simulink model "BlueRov2PID"  (R2025a)
settings: Solver=ode4  StartTime=0.0  StopTime=30  FixedStep=0.001  RelTol=1e-3
settings Model: Creator=oisin  LastModifiedBy=oisin
settings DataIOCC: ReturnWorkspaceOutputsName=PID

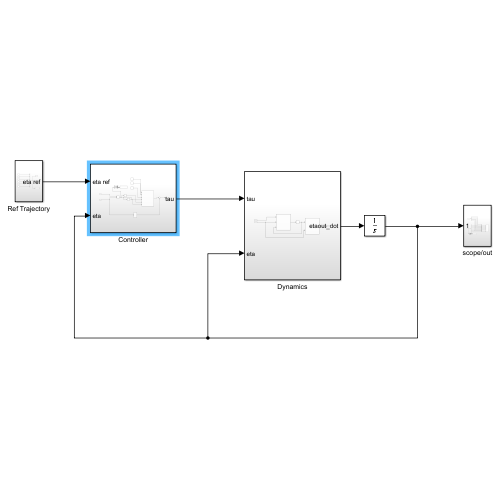
[thumbnail: Simulink's stored preview of the top-level diagram]
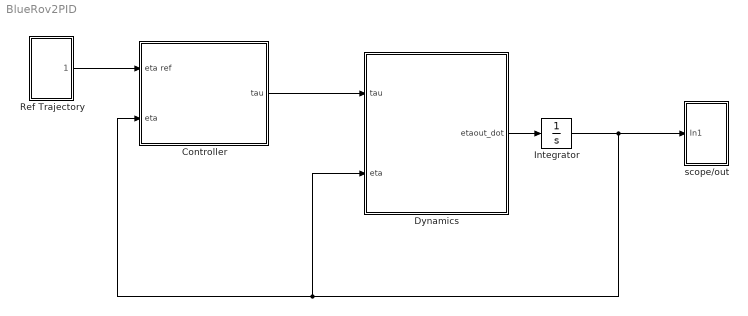
== system BlueRov2PID ==
  Controller : Subsystem
  Dynamics : Subsystem
  Integrator : Integrator  InitialCondition=[10;0;0;0;0;0]
  Ref Trajectory : Subsystem
  scope/out : Subsystem
  wires:
  Ref Trajectory/1(eta ref) -> Controller/1(eta ref)
  Integrator/1 -> Dynamics/2(eta), Controller/2(eta), scope/out/1(In1)
  Controller/1(tau) -> Dynamics/1(tau)
  Dynamics/1(etaout_dot) -> Integrator/1

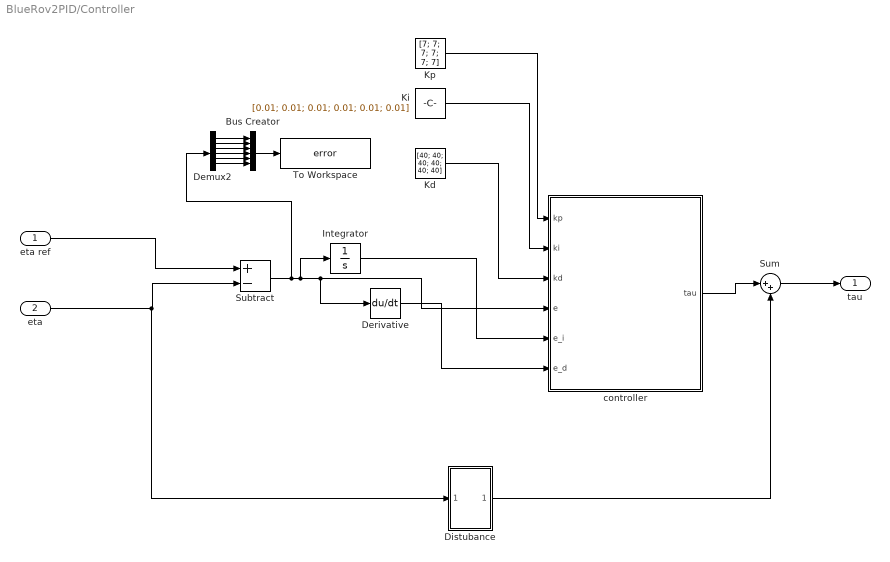
== system BlueRov2PID/Controller ==
  eta ref : Inport
  eta : Inport  Port=2
  Bus Creator : BusCreator  Inputs=6
  Demux2 : Demux  Outputs=6
  Derivative : Derivative
  Distubance : Subsystem
  Integrator : Integrator
  Kd : Constant  Value=[40; 40; 40; 40; 40; 40]
  Ki : Constant  Value=[0.01; 0.01; 0.01; 0.01; 0.01; 0.01]
  Kp : Constant  Value=[7; 7; 7; 7; 7; 7]
  Subtract : Sum  Inputs=+-
  Sum : Sum  Inputs=|++
  To Workspace : ToWorkspace  VariableName=error  SampleTime=-1
  controller : MATLAB Function  TreatAsAtomicUnit=on
  tau : Outport
  wires:
  eta/1 -> Distubance/1(eta), Subtract/2
  eta ref/1 -> Subtract/1
  Subtract/1 -> Demux2/1, Derivative/1, controller/4(e), Integrator/1
  Derivative/1 -> controller/6(e_d)
  Integrator/1 -> controller/5(e_i)
  controller/1(tau) -> Sum/1
  Sum/1 -> tau/1
  Kp/1 -> controller/1(kp)
  Ki/1 -> controller/2(ki)
  Kd/1 -> controller/3(kd)
  Distubance/1(Out1) -> Sum/2
  Demux2/3 -> Bus Creator/3
  Demux2/2 -> Bus Creator/2
  Demux2/1 -> Bus Creator/1
  Demux2/4 -> Bus Creator/4
  Bus Creator/1 -> To Workspace/1
  Demux2/5 -> Bus Creator/5
  Demux2/6 -> Bus Creator/6

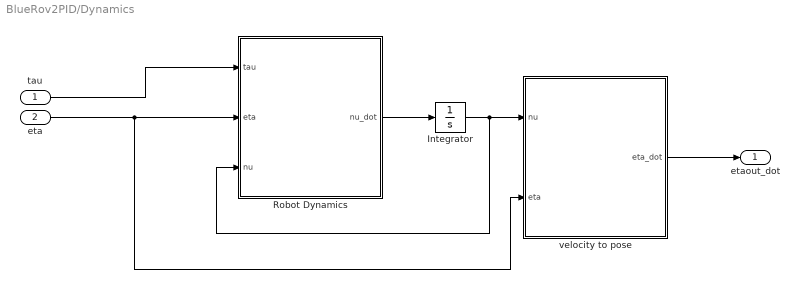
== system BlueRov2PID/Dynamics ==
  tau : Inport
  eta : Inport  Port=2
  Integrator : Integrator
  Robot Dynamics : MATLAB Function  TreatAsAtomicUnit=on
  velocity to pose : MATLAB Function  TreatAsAtomicUnit=on
  etaout_dot : Outport
  wires:
  Robot Dynamics/1(nu_dot) -> Integrator/1
  tau/1 -> Robot Dynamics/1(tau)
  eta/1 -> velocity to pose/2(eta), Robot Dynamics/2(eta)
  Integrator/1 -> Robot Dynamics/3(nu), velocity to pose/1(nu)
  velocity to pose/1(eta_dot) -> etaout_dot/1

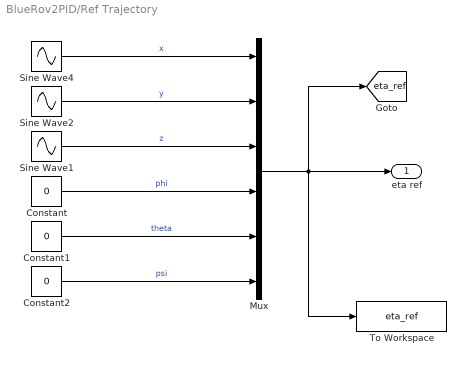
== system BlueRov2PID/Ref Trajectory ==
  Constant : Constant  Value=0
  Constant1 : Constant  Value=0
  Constant2 : Constant  Value=0
  Mux : Mux  Inputs=6
  Sine Wave1 : Sin  Amplitude=5  Bias=-10  Frequency=pi/6  Phase=pi/2  SampleTime=0
  Sine Wave2 : Sin  Amplitude=10  Frequency=(2*pi)/30  SampleTime=0
  Sine Wave4 : Sin  Amplitude=10  Frequency=(2*pi)/30  Phase=pi/2  SampleTime=0
  To Workspace : ToWorkspace  VariableName=eta_ref  SaveFormat=Timeseries  SampleTime=-1
  eta ref : Outport
  tag scope: eta_ref=global
  wires:
  Constant/1 -> Mux/4  "phi"
  Constant1/1 -> Mux/5  "theta"
  Sine Wave4/1 -> Mux/1  "x"
  Constant2/1 -> Mux/6  "psi"
  Mux/1 -> To Workspace/1, [eta_ref], eta ref/1
  Sine Wave2/1 -> Mux/2  "y"
  Sine Wave1/1 -> Mux/3  "z"

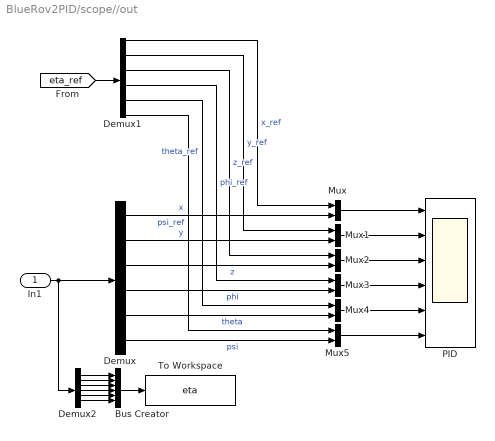
== system BlueRov2PID/scope//out ==
  In1 : Inport
  Bus Creator : BusCreator  Inputs=6
  Demux : Demux  Outputs=6
  Demux1 : Demux  Outputs=6
  Demux2 : Demux  Outputs=6
  Mux{,1..5} (6 alike) : Mux  Inputs=2
  PID : Scope  NumInputPorts=6
      settings: ActiveDisplayYMinimum=-12.5055733321088  ActiveDisplayYMaximum=12.550159988979194
  To Workspace : ToWorkspace  VariableName=eta  SampleTime=-1
  wires:
  Mux5/1 -> PID/6
  Mux/1 -> PID/1
  Demux/4 -> Mux3/2  "phi"
  Demux/6 -> Mux5/2  "psi"
  Demux/3 -> Mux2/2  "z"
  Mux3/1 -> PID/4
  Demux/5 -> Mux4/2  "theta"
  Mux1/1 -> PID/2
  Demux/1 -> Mux/2  "x"
  Demux1/4 -> Mux3/1  "phi_ref"
  Demux1/3 -> Mux2/1  "z_ref"
  Demux1/2 -> Mux1/1  "y_ref"
  Demux1/1 -> Mux/1  "x_ref"
  Demux/2 -> Mux1/2  "y"
  [eta_ref] -> Demux1/1
  Mux2/1 -> PID/3
  Mux4/1 -> PID/5
  Demux1/6 -> Mux5/1  "psi_ref"
  Demux1/5 -> Mux4/1  "theta_ref"
  In1/1 -> Demux2/1, Demux/1
  Demux2/1 -> Bus Creator/1
  Demux2/2 -> Bus Creator/2
  Demux2/3 -> Bus Creator/3
  Demux2/4 -> Bus Creator/4
  Demux2/5 -> Bus Creator/5
  Demux2/6 -> Bus Creator/6
  Bus Creator/1 -> To Workspace/1

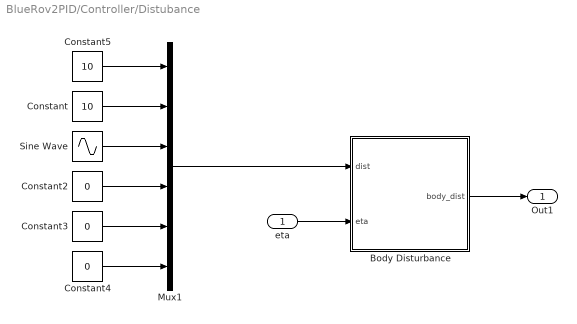
== system BlueRov2PID/Controller/Distubance ==
  eta : Inport
  Body Disturbance : MATLAB Function  TreatAsAtomicUnit=on
  Constant : Constant  Value=10
  Constant2 : Constant  Value=0
  Constant3 : Constant  Value=0
  Constant4 : Constant  Value=0
  Constant5 : Constant  Value=10
  Mux1 : Mux  Inputs=6
  Sine Wave : Sin  Amplitude=10  SampleTime=0
  Out1 : Outport
  wires:
  Constant2/1 -> Mux1/4
  Constant3/1 -> Mux1/5
  Constant4/1 -> Mux1/6
  Body Disturbance/1(body_dist) -> Out1/1
  Mux1/1 -> Body Disturbance/1(dist)
  eta/1 -> Body Disturbance/2(eta)
  Constant5/1 -> Mux1/1
  Constant/1 -> Mux1/2
  Sine Wave/1 -> Mux1/3

== matlab function BlueRov2PID/Dynamics/velocity to pose ==
  data: nu input; eta_dot output; eta input
function eta_dot = fcn(nu, eta)

eta_dot=zeros(6,1);

x=eta(1,1);
y=eta(2,1);
z=eta(3,1);
phi=eta(4,1);
theta=eta(5,1);
psi=eta(6,1);

J=[(cos(psi)*(cos(theta))),((-sin(psi))*(cos(phi)))+((cos(psi))*(sin(theta))*(sin(phi))),((sin(psi))*(sin(phi)))+((cos(psi))*(cos(phi))*(sin(theta))),0,0,0;
    (sin(psi))*(cos(theta)),((cos(psi))*(cos(phi)))+((sin(phi))*(sin(theta))*(sin(psi))),((-cos(psi))*(sin(phi)))+((sin(theta))*(sin(psi))*(cos(phi))),0,0,0;
    -sin(theta),(cos(theta))*(sin(phi)),(cos(theta))*(cos(phi)),0,0,0;
    0,0,0,1,(sin(phi))*(tan(theta)),(cos(phi))*(tan(theta));
    0,0,0,0,cos(phi),-sin(phi);
    0,0,0,0,(sin(phi))/(cos(theta)),(cos(phi))/(cos(theta))];

eta_dot = J * nu;

== matlab function BlueRov2PID/Dynamics/Robot Dynamics ==
  data: tau input; nu_dot output; eta input; nu input
function nu_dot = fcn(tau, eta, nu)

nu_dot=zeros(6,1);

t1=tau(1,1);
t2=tau(2,1);
t3=tau(3,1);
t4=tau(4,1);
t5=tau(5,1);
t6=tau(6,1);

tautot=[t1;t2;t3;t4;t5;t6];

m  = 11.5;
W  = 112.8;
B  = 114.8;

Ix = 0.16;
Iy = 0.16;
Iz = 0.16;
zg = 0.0;

X_udot  = -5.5;
Y_vdot  = -12.7;
Z_wdot  = -14.57;
K_pdot  = -0.12;
M_qdot  = -0.12;
N_rdot  = -0.12; 

X_u = -4.03;
Y_v = -6.22;
Z_w = -5.18;
K_p = -0.07;
M_q = -0.07;
N_r = -0.07;

X_uu        = -18.18;
Y_vv        = -21.66;
Z_ww        = -36.99;
K_pp        = -1.55;
M_qq        = -1.55; 
N_rr        = -1.55;  

x=eta(1,1);
y=eta(2,1);
z=eta(3,1);
phi=eta(4,1);
theta=eta(5,1);
psi=eta(6,1);

J=[(cos(psi)*(cos(theta))),((-sin(psi))*(cos(phi)))+((cos(psi))*(sin(theta))*(sin(phi))),((sin(psi))*(sin(phi)))+((cos(psi))*(cos(phi))*(sin(theta))),0,0,0;
    (sin(psi))*(cos(theta)),((cos(psi))*(cos(phi)))+((sin(phi))*(sin(theta))*(sin(psi))),((-cos(psi))*(sin(phi)))+((sin(theta))*(sin(psi))*(cos(phi))),0,0,0;
    -sin(theta),(cos(theta))*(sin(phi)),(cos(theta))*(cos(phi)),0,0,0;
    0,0,0,1,(sin(phi))*(tan(theta)),(cos(phi))*(tan(theta));
    0,0,0,0,cos(phi),-sin(phi);
    0,0,0,0,(sin(phi))/(cos(theta)),(cos(phi))/(cos(theta))];

u=nu(1,1);
v=nu(2,1);
w=nu(3,1);
p=nu(4,1);
q=nu(5,1);
r=nu(6,1);

% mass matrices
M_A = -diag([X_udot,Y_vdot,Z_wdot,K_pdot,M_qdot,N_rdot]);

M_RB = [ m   0    0    0      m*zg  0;
          0   m    0   -m*zg   0     0;
          0   0    m    0      0     0;
          0  -m*zg 0   Ix      0     0;
          m*zg 0   0    0      Iy    0;
          0    0   0    0      0     Iz ];


M_total = M_A + M_RB;

% coriolis matrices
C_A = [ 0     0     0      0          Z_wdot*w     0;
         0     0     0     -Z_wdot*w  0            -X_udot*u;
         0     0     0      Y_vdot*v   -N_rdot*r    0;
         0     Z_wdot*w  -Y_vdot*v    0            -K_pdot*p   0;
        -Z_wdot*w   0     X_udot*u    K_pdot*p      0          0;
        -Y_vdot*v  X_udot*u   0       0             0          0 ];

C_RB = [ 0     0     0     0     m*w   -m*v;
          0     0     0    -m*w   0      m*u;
          0     0     0     m*v  -m*u    0;
          0    -m*w   m*v   0    Iz*r   -Iy*q;
          m*w   0    -m*u  -Iz*r 0       Ix*p;
         -m*v   m*u   0     Iy*q -Ix*p   0 ];

C_total = C_A + C_RB;

% restoring forces
g_eta = [ (W - B) * sin(theta);
         -(W - B) * cos(theta) * sin(phi);
         -(W - B) * cos(theta) * cos(phi);
          zg * W * cos(theta) * sin(phi);
          zg * W * sin(theta);
          0 ];

% damping
D_lin = -diag([X_u, Y_v, Z_w, K_p, M_q, N_r]);

D_quad = -diag([X_uu*abs(u), Y_vv*abs(v), Z_ww*abs(w), K_pp*abs(p), M_qq*abs(q), N_rr*abs(r)]);

D_total = D_lin + D_quad;

% calculate nu_dot
nu_dot = M_total \ (tautot-((C_total*nu)+(D_total*nu)+g_eta));

== matlab function BlueRov2PID/Controller/controller ==
  data: kp input; ki input; kd input; tau output; e input; e_i input; e_d input
function tau = fcn(kp, ki, kd, e,e_i,e_d)

% Define limits
max_tau = [88; 88; 137; 23.3; 23.3; 21.6];
tau_unsat = kp .* e + ki .* e_i + kd .* e_d;
%Saturated
tau = max(min(tau_unsat, max_tau), -max_tau);

%tau = kp .* e + ki .* e_i + kd .* e_d;

== matlab function BlueRov2PID/Controller/Distubance/Body Disturbance ==
  data: dist input; body_dist output; eta input
function body_dist  = fcn(dist,eta)

phi=eta(4,1);
theta=eta(5,1);
psi=eta(6,1);

J=[(cos(psi)*(cos(theta))),((-sin(psi))*(cos(phi)))+((cos(psi))*(sin(theta))*(sin(phi))),((sin(psi))*(sin(phi)))+((cos(psi))*(cos(phi))*(sin(theta))),0,0,0;
    (sin(psi))*(cos(theta)),((cos(psi))*(cos(phi)))+((sin(phi))*(sin(theta))*(sin(psi))),((-cos(psi))*(sin(phi)))+((sin(theta))*(sin(psi))*(cos(phi))),0,0,0;
    -sin(theta),(cos(theta))*(sin(phi)),(cos(theta))*(cos(phi)),0,0,0;
    0,0,0,1,(sin(phi))*(tan(theta)),(cos(phi))*(tan(theta));
    0,0,0,0,cos(phi),-sin(phi);
    0,0,0,0,(sin(phi))/(cos(theta)),(cos(phi))/(cos(theta))];


body_dist= J \ dist;
